simulink model "Orbit_Propagator"  (R2022b)
settings: Solver=ode4  StartTime=0  StopTime=time_end  FixedStep=time_step  RelTol=1e-9  AbsTol=1e-9
undefined symbols (not defined in the file or in its folder): COE_chaser, COE_target, Constants, PropOptions
settings Model: Creator=Cory  LastModifiedBy=coryt
settings SolverCC: AlgebraicLoopSolver=TrustRegion
settings DataIOCC: ReturnWorkspaceOutputs=off
settings DebuggingCC: UnconnectedInputMsg=warning  UnconnectedOutputMsg=warning  UnconnectedLineMsg=warning  SFMachineParentedDataDiag=warning  ArithmeticOperatorsInVariantConditions=warning
settings ModelReferenceCC: EnableRefExpFcnMdlSchedulingChecks=on
settings SFSimCC: SimUseLocalCustomCode=off  CustomCodeUndefinedFunction=UseInterfaceOnly
settings RTWCC: RTWUseLocalCustomCode=off

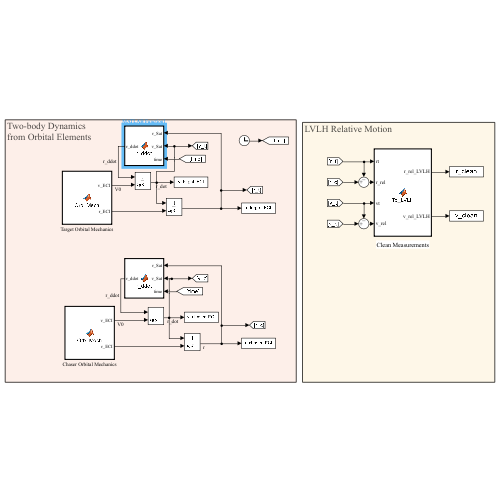
[thumbnail: Simulink's stored preview of the top-level diagram]
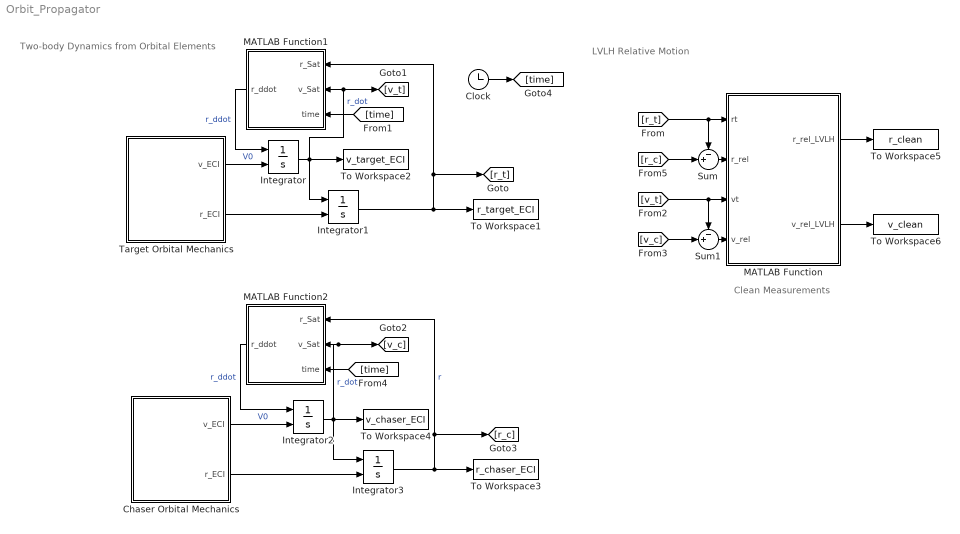
== system Orbit_Propagator ==
  note: LVLH Relative Motion
  note: Two-body Dynamics
      | from Orbital Elements
  note: Clean Measurements
  Chaser Orbital Mechanics : MATLAB Function  TreatAsAtomicUnit=on
  Clock : Clock
  Integrator{,1..3} (4 alike) : Integrator  InitialConditionSource=external
  MATLAB Function : MATLAB Function  TreatAsAtomicUnit=on
  MATLAB Function1 : MATLAB Function  TreatAsAtomicUnit=on
  MATLAB Function2 : MATLAB Function  TreatAsAtomicUnit=on
  Sum : Sum  Inputs=-+|
  Sum1 : Sum  Inputs=-+|
  Target Orbital Mechanics : MATLAB Function  TreatAsAtomicUnit=on
  To Workspace1 : ToWorkspace  VariableName=r_target_ECI  SampleTime=-1
  To Workspace2 : ToWorkspace  VariableName=v_target_ECI  SampleTime=-1
  To Workspace3 : ToWorkspace  VariableName=r_chaser_ECI  SampleTime=-1
  To Workspace4 : ToWorkspace  VariableName=v_chaser_ECI  SampleTime=-1
  To Workspace5 : ToWorkspace  VariableName=r_clean  SampleTime=-1
  To Workspace6 : ToWorkspace  VariableName=v_clean  SampleTime=-1
  wires:
  Target Orbital Mechanics/1(v_ECI) -> Integrator/2  "V0"
  MATLAB Function1/1(r_ddot) -> Integrator/1  "r_ddot"
  Integrator/1 -> [v_t], MATLAB Function1/2(v_Sat), To Workspace2/1, Integrator1/1  "r_dot"
  Integrator1/1 -> [r_t], MATLAB Function1/1(r_Sat), To Workspace1/1
  Target Orbital Mechanics/2(r_ECI) -> Integrator1/2
  Chaser Orbital Mechanics/1(v_ECI) -> Integrator2/2  "V0"
  Chaser Orbital Mechanics/2(r_ECI) -> Integrator3/2
  Integrator3/1 -> To Workspace3/1, [r_c], MATLAB Function2/1(r_Sat)  "r"
  MATLAB Function2/1(r_ddot) -> Integrator2/1  "r_ddot"
  Integrator2/1 -> [v_c], MATLAB Function2/2(v_Sat), To Workspace4/1, Integrator3/1  "r_dot"
  MATLAB Function/2(v_rel_LVLH) -> To Workspace6/1
  [v_c] -> Sum1/2
  [r_t] -> Sum/1, MATLAB Function/1(rt)
  Sum1/1 -> MATLAB Function/4(v_rel)
  [r_c] -> Sum/2
  Sum/1 -> MATLAB Function/2(r_rel)
  [v_t] -> Sum1/1, MATLAB Function/3(vt)
  MATLAB Function/1(r_rel_LVLH) -> To Workspace5/1
  Clock/1 -> [time]
  [time] -> MATLAB Function1/3(time)
  [time] -> MATLAB Function2/3(time)

== matlab function Orbit_Propagator/MATLAB Function ==
  data: rt input; r_rel input; vt input; r_rel_LVLH output; v_rel input; v_rel_LVLH output
 function [r_rel_LVLH, v_rel_LVLH] = To_LVLH(rt, r_rel, vt, v_rel)
% =========================================================================
% Description: This function converts the relative r and v from ECI Frame
% to LVLH Frame by applying the appropriate rotation matrices.
% =========================================================================
%Determine unit vectors for LVLH Frame
Lx      = rt/norm(rt);
Lz      = cross(rt, vt)/norm(cross(rt, vt));
Ly      = cross(Lz, Lx);

%Align unit vectors into rows
Lx      = Lx';
Ly      = Ly';
Lz      = Lz';

%Arranging vectrix for LVLH Frame
F_LVLH  = [ Lx      
            Ly
            Lz ];

%ECI Frame is defined as such
F_ECI   = [ 1 0 0 
            0 1 0
            0 0 1 ];
     
%Compute roration matrix - ECI to LVLH
C_LI    = F_LVLH*F_ECI';

%Computing relative velocity in LVLH frame, accounting for rotation 
omega =  cross(rt,vt)/norm(rt)^2;
v_rel = v_rel - cross(omega,r_rel);

%Apply rotation to obtain relative LVLH parameters
r_rel_LVLH = C_LI*r_rel; 
v_rel_LVLH = C_LI*v_rel;

end
% =========================================================================

== matlab function Orbit_Propagator/MATLAB Function2 ==
  data: r_Sat input; r_ddot output; v_Sat input; Constants parameter; PropOptions parameter; time input
function r_ddot = r_ddot(r_Sat, v_Sat, Constants, PropOptions, time)
% ========================================================================
% Description: This function calculates -mu/r^3 *r to propagate the radius
% vector of the orbital motion

coder.extrinsic('Accelerations');

r_ddot = zeros(3,1);
r_ddot = Accelerations(r_Sat, v_Sat, Constants, PropOptions, time);

end
% ========================================================================

== matlab function Orbit_Propagator/Chaser Orbital Mechanics ==
  data: COE_chaser parameter; v_ECI output; r_ECI output; Constants parameter
function [v_ECI,r_ECI] = Orb_Mech(COE_chaser, Constants)
% ========================================================================
% Description: This funciton calculates the initial r and v vectors, 
% given the provided classiclal orbital elements defined in the
% initialization of the simulation.

%%========================================================================
%Extract COE values
theta       = COE_chaser(1);
a           = COE_chaser(2);
e           = COE_chaser(3);
i           = COE_chaser(4);
RAAN        = COE_chaser(5);
w           = COE_chaser(6);

mu = Constants.mu_Earth;
%%========================================================================
r   = a*(1-e^2)/(1+e*cos(theta));                               %Defining the radius (Eq. 2.32)
p   = a*(1-e^2);                                                %Defining the semilatus rectum (Eq. 31)
r_P = [r*cos(theta) r*sin(theta) 0]';                           %(r in perifocal frame - Eq. 2.86) 
v_P = [-sqrt(mu/p)*sin(theta) sqrt(mu/p)*(e+cos(theta)) 0]';    %(v in perifocal frame - Eq. 2.87)

%Rotation Matrix from P to ECI Frame
C_IP = [    cos(RAAN)*cos(w)-sin(RAAN)*cos(i)*sin(w) -cos(RAAN)*sin(w)-sin(RAAN)*cos(i)*cos(w) sin(RAAN)*sin(i);
            sin(RAAN)*cos(w)+cos(RAAN)*cos(i)*sin(w) -sin(RAAN)*sin(w)+cos(RAAN)*cos(i)*cos(w) -cos(RAAN)*sin(i);
                        sin(i)*sin(w)                            sin(i)*cos(w)                       cos(i)  ];

%Definition of ECI Frame
x_ECI   = [1 0 0];
y_ECI   = [0 1 0];
z_ECI   = [0 0 1];
F_ECI   = [x_ECI; y_ECI; z_ECI]; %Reference Frame ECI

%r and v vectors in ECI Frame
r_ECI   = F_ECI*C_IP*r_P;
v_ECI   = F_ECI*C_IP*v_P;

%z_vec_ECI  = cross(r_ECI, v_ECI)/norm(cross(r_ECI, v_ECI));    %Check orientation of z vector
%X_ECI      = [r_ECI v_ECI]';                                   %State Vector in ECI components (Eq. 2.82)

r_mag = norm(r_ECI);
r_hat = r_ECI/r_mag;

end
% ========================================================================

== matlab function Orbit_Propagator/MATLAB Function1 ==
  data: r_Sat input; v_Sat input; r_ddot output; Constants parameter; PropOptions parameter; time input
function r_ddot = r_ddot(r_Sat, v_Sat, Constants, PropOptions, time)
% ========================================================================
% Description: This function calculates -mu/r^3 *r to propagate the radius
% vector of the orbital motion

coder.extrinsic('Accelerations');

r_ddot = zeros(3,1);
r_ddot = Accelerations(r_Sat, v_Sat, Constants, PropOptions, time);

end
% ========================================================================

== matlab function Orbit_Propagator/Target Orbital Mechanics ==
  data: COE_target parameter; v_ECI output; r_ECI output; Constants parameter
 function [v_ECI,r_ECI] = Orb_Mech(COE_target, Constants)
% ========================================================================
% Description: This funciton calculates the initial r and v vectors, 
% given the provided classiclal orbital elements defined in the
% initialization of the simulation.

%%========================================================================
%Extract COE values
theta       = COE_target(1);
a           = COE_target(2);
e           = COE_target(3);
i           = COE_target(4);
RAAN        = COE_target(5);
w           = COE_target(6);

mu_Earth = Constants.mu_Earth;
%%========================================================================
r   = a*(1-e^2)/(1+e*cos(theta));                               %Defining the radius (Eq. 2.32)
p   = a*(1-e^2);                                                %Defining the semilatus rectum (Eq. 2.31)
r_P = [r*cos(theta) r*sin(theta) 0]';                           %(r in perifocal frame - Eq. 2.86) 
v_P = [-sqrt(mu_Earth/p)*sin(theta) sqrt(mu_Earth/p)*(e+cos(theta)) 0]';    %(v in perifocal frame - Eq. 2.87)

%Rotation Matrix from P to ECI Frame
C_IP = [    cos(RAAN)*cos(w)-sin(RAAN)*cos(i)*sin(w) -cos(RAAN)*sin(w)-sin(RAAN)*cos(i)*cos(w) sin(RAAN)*sin(i);
            sin(RAAN)*cos(w)+cos(RAAN)*cos(i)*sin(w) -sin(RAAN)*sin(w)+cos(RAAN)*cos(i)*cos(w) -cos(RAAN)*sin(i);
                        sin(i)*sin(w)                            sin(i)*cos(w)                       cos(i)  ];

%Definition of ECI Frame
x_ECI   = [1 0 0];
y_ECI   = [0 1 0];
z_ECI   = [0 0 1];
F_ECI   = [x_ECI; y_ECI; z_ECI]; %Reference Frame ECI

%r and v vectors in ECI Frame
r_ECI   = F_ECI*C_IP*r_P;
v_ECI   = F_ECI*C_IP*v_P;

%z_vec_ECI  = cross(r_ECI, v_ECI)/norm(cross(r_ECI, v_ECI));    %Check orientation of z vector
%X_ECI      = [r_ECI v_ECI]';                                   %State Vector in ECI components (Eq. 2.82)

r_mag = norm(r_ECI);
r_hat = r_ECI/r_mag;

end
% ========================================================================
